simulink model "Disco_Resorte"  (R2022b)
settings: Solver=VariableStepAuto  StartTime=0.0  StopTime=10  MaxStep=0.0003  RelTol=1e-3
values from neighbouring files (symbols this model uses):
  k = 100    [DiscoResorte.m]    (also in parametros_disco_resorte.m)
  m = 10    [DiscoResorte.m]    (also in parametros_disco_resorte.m)
  r = 0.05    [DiscoResorte.m]    (also in parametros_disco_resorte.m)
libraries: fl_lib x6, nesl_utility x2
settings Model: Creator=jesus  LastModifiedBy=jesus

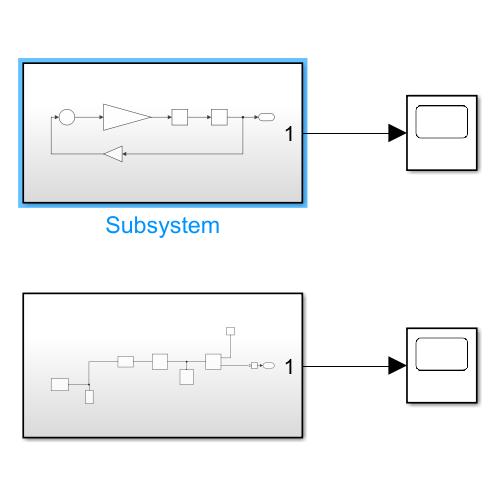
[thumbnail: Simulink's stored preview of the top-level diagram]
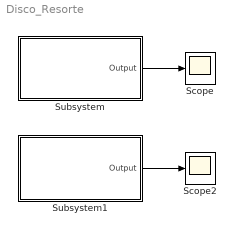
== system Disco_Resorte ==
  Scope : Scope
  Scope2 : Scope
  Subsystem : Subsystem
  Subsystem1 : Subsystem
  wires:
  Subsystem/1(Output) -> Scope/1
  Subsystem1/1(Output) -> Scope2/1

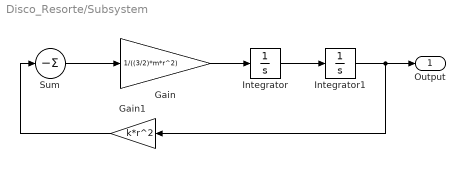
== system Disco_Resorte/Subsystem ==
  Gain : Gain  Gain=1/((3/2)*m*r^2)
  Gain1 : Gain  Gain=k*r^2
  Integrator : Integrator  InitialCondition=2
  Integrator1 : Integrator
  Sum : Sum  Inputs=-
  Output : Outport
  wires:
  Integrator/1 -> Integrator1/1
  Sum/1 -> Gain/1
  Integrator1/1 -> Output/1, Gain1/1
  Gain/1 -> Integrator/1
  Gain1/1 -> Sum/1

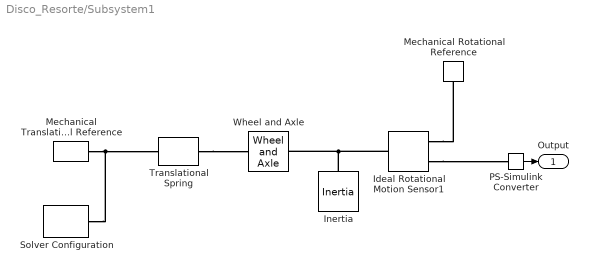
== system Disco_Resorte/Subsystem1 ==
  Ideal Rotational Motion Sensor1 : fl_lib/Mechanical/Mechanical Sensors/Ideal Rotational Motion Sensor  reference=foundation.enum.MeasurementReference.difference  acceleration_port=false  velocity_port=false  position_port=true  wrap_angle=false  offset=0 rad
      settings: InternalSimscapePortConfiguration="{\"Bottom\":[],\"Left\":[{\"id\":\"R\",\"label\":\"R\",\"type\":\"foundation.mechanical.rotational.rotational\"}],\"Right\":[{\"id\":\"C\",\"label\":\"C\",\"type\":\"foundation.mechanical.rotational.rotational\"},{\"id\":\"A\",\"label\":\"A\",\"type\":\"output\"}],\"Top\":[]}"
  Inertia : fl_lib/Mechanical/Rotational Elements/Inertia  inertia=0.0375 kg*m^2  num_ports=foundation.enum.numPorts2.one  w_specify=on  w_priority=High  w=2 rad/s  w_nominal_specify=off  w_nominal_unit=rad/s  w_nominal_value=1  t_specify=off  t_priority=None  t=0 N*m  t_nominal_specify=off  t_nominal_unit=N*m  t_nominal_value=1
  Mechanical Rotational Reference : fl_lib/Mechanical/Rotational Elements/Mechanical Rotational Reference
  Mechanical Translational Reference : fl_lib/Mechanical/Translational Elements/Mechanical Translational Reference
  PS-Simulink Converter : nesl_utility/PS-Simulink Converter  PhysicalDomain=network_engine_domain  SubClassName=ps_output  LeftPortType=input  RightPortType=output  PseudoPeriodic=off  Frequencies=[]  VectorFormat=inherit  Unit=inherit  AffineConversion=off
  Solver Configuration : nesl_utility/Solver Configuration  PhysicalDomain=network_engine_domain  SubClassName=solver  LeftPortType=input  RightPortType=generic  Tones=[]  Harmonics=[]  SimulateNoise=off  Profile=off  UseLocalSampling=off  EnableSwitchedLinearOptims=on  FrequencyDomain=off  UseCCode=off  RelTol=0.001  AbsTol=0.001  MinStep=1e-09  ToWorkspace=off  RevertToSquareIcSolve=off  NumHomotopyIterations=100  PhasorMode=off  PhasorModeNumHarmonics=1  ConsistencySolver=NEWTON_XTOL_AFTER_FTOL  IndexReductionMethod=DerivativeReplacement  DoDC=off  ResidualTolerance=1e-09  ConsistencyTolSource=GLOBAL  ConsistencyAbsTol=0.001  ConsistencyRelTol=0.001  ConsistencyTolFactor=0.001  UseLocalSolver=off  LocalSolverChoice=NE_BACKWARD_EULER_ADVANCER  ResolveIndetEquations=on  FunctionEvalNumThread=1  LocalSolverSampleTime=0.001  DoFixedCost=off  MaxNonlinIter=3  MaxModeIter=2  ComputeImpulses=off  ImpulseIterations=2  LinearAlgebra=auto  LinearAlgebraNumThread=0  EquationFormulation=NE_TIME_EF  DelaysMemoryBudget=1024  AutomaticFiltering=on  FilteringTimeConstant=0.001  PartitionStorageMethod=AS_NEEDED  PartitionMemoryBudget=1024  PartitionMethod=ROBUST
  Translational Spring : fl_lib/Mechanical/Translational Elements/Translational Spring  spr_rate=100 N/m  v_specify=off  v_priority=None  v=0 m/s  v_nominal_specify=off  v_nominal_unit=m/s  v_nominal_value=1  f_specify=off  f_priority=None  f=0 N  f_nominal_specify=off  f_nominal_unit=N  f_nominal_value=1  x_specify=off  x_priority=High  x=0 m  x_nominal_specify=off  x_nominal_unit=m  x_nominal_value=1
  Wheel and Axle : fl_lib/Mechanical/Mechanisms/Wheel and Axle  R=0.05 m  or=1  t_specify=off  t_priority=None  t=0 N*m  t_nominal_specify=off  t_nominal_unit=N*m  t_nominal_value=1  f_specify=off  f_priority=None  f=0 N  f_nominal_specify=off  f_nominal_unit=N  f_nominal_value=1
  Output : Outport
  wires:
  PS-Simulink Converter/1 -> Output/1
  connections:
  Ideal Rotational Motion Sensor1/LConn1 -- Wheel and Axle/LConn1 -- Inertia/LConn1
  Translational Spring/RConn1 -- Wheel and Axle/RConn1
  Ideal Rotational Motion Sensor1/RConn1 -- Mechanical Rotational Reference/LConn1
  Ideal Rotational Motion Sensor1/RConn2 -- PS-Simulink Converter/LConn1
  Mechanical Translational Reference/LConn1 -- Solver Configuration/RConn1 -- Translational Spring/LConn1
